simulink model "Simulation"  (R2022b)
settings: Solver=FixedStepAuto  StartTime=0.0  StopTime=param.Tsim  FixedStep=param.tSample  RelTol=1e-3
StopFcn:
  | run animation
  | run plotSol
undefined symbols (not defined in the file or in its folder): f, filterFr, filterFw, filterMr, FR_neg, FR_pos, g1, g2, g3, kFr, ki, kiSeil, kMr, kp, kpSeil, kVSl, kVSx, MR, MRP, param, xi_0
libraries: simulink x10, spsFirstOrderFilterLib x2
(part 2 of 3)

== system Simulation/Flatness-based control1/dynamic tracking control/Computation of the flat output ==
  Control input : Inport
  States : Inport  Port=2
  Demux : Demux  Outputs=8
  Demux1 : Demux  Outputs=2
  Derivative : Derivative
  Derivative1 : Derivative
  MATLAB Function : MATLAB Function  TreatAsAtomicUnit=on
  MATLAB Function1 : MATLAB Function  TreatAsAtomicUnit=on
  MATLAB Function2 : MATLAB Function  TreatAsAtomicUnit=on
  Mux : Mux
  Mux1 : Mux
  z1_xLoad : Outport
  z2_yLoad : Outport  Port=2
  wires:
  MATLAB Function/2(z2) -> Mux1/1
  Derivative/1 -> Mux/4
  MATLAB Function2/1(ddz1) -> Mux/3, Derivative/1
  MATLAB Function/1(z1) -> Mux/1
  Demux/2 -> MATLAB Function1/1(x2)
  Demux/6 -> MATLAB Function2/3(x6), MATLAB Function1/5(x6)
  MATLAB Function2/2(ddz2) -> Mux1/3, Derivative1/1
  Control input/1 -> Demux1/1
  MATLAB Function1/2(dz2) -> Mux1/2
  Demux/5 -> MATLAB Function/3(x5), MATLAB Function2/2(x5), MATLAB Function1/4(x5)
  Demux/1 -> MATLAB Function/1(x1)
  States/1 -> Demux/1
  Demux/3 -> MATLAB Function2/1(x3), MATLAB Function1/2(x3), MATLAB Function/2(x3)
  Demux/4 -> MATLAB Function1/3(x4)
  MATLAB Function1/1(dz1) -> Mux/2
  Derivative1/1 -> Mux1/4
  Mux/1 -> z1_xLoad/1
  Mux1/1 -> z2_yLoad/1
  Demux1/1 -> MATLAB Function2/4(u1)
  Demux1/2 -> MATLAB Function2/5(u2)

== system Simulation/Flatness-based control1/dynamic tracking control/System extension ==
  u_extended : Inport
  x_real : Inport  Port=2
  Demux : Demux  Outputs=6
  Demux1 : Demux  Outputs=2
  Integrator : Integrator
  Integrator1 : Integrator
  MATLAB Function3 : MATLAB Function  TreatAsAtomicUnit=on
  Mux : Mux  Inputs=8
  u2_real : Outport
  x_extended : Outport  Port=2
  wires:
  u_extended/1 -> Demux1/1
  x_real/1 -> Demux/1
  Mux/1 -> x_extended/1
  Demux/1 -> Mux/1
  Demux1/1 -> MATLAB Function3/5(u1_ext), Mux/2
  Demux/3 -> Mux/3, MATLAB Function3/2(x3)
  MATLAB Function3/1(u2_real) -> Mux/4, u2_real/1
  Demux/5 -> MATLAB Function3/3(x5), Mux/5
  Demux/6 -> Mux/6, MATLAB Function3/4(x6)
  Demux1/2 -> Integrator/1
  Integrator/1 -> Mux/8, Integrator1/1  "x2_ext"
  Integrator1/1 -> Mux/7, MATLAB Function3/1(x1_ext)  "x1_ext"

== system Simulation/Flatness-based control1/dynamic tracking control/Tracking controller ==
  z1_xLoad : Inport
  z2_yLoad : Inport  Port=2
  z1_d_xLoad : Inport  Port=3
  z2_d_yLoad : Inport  Port=4
  Constant : Constant  Value=[param.pX01 param.pX02 param.pX03 param.pX04]
  Constant1 : Constant  Value=[param.pY01_DYN param.pY02_DYN param.pY03_DYN param.pY04_DYN]
  Demux : Demux
  Demux1 : Demux
  MATLAB Function : MATLAB Function  TreatAsAtomicUnit=on
  Tracking controller v1 for xLoad : Subsystem
  Tracking controller v2 for yLoad : Subsystem
  u1_aCart : Outport
  u2_aRope : Outport  Port=2
  wires:
  Constant1/1 -> Tracking controller v2 for yLoad/3(Koeffizienten2)
  Constant/1 -> Tracking controller v1 for xLoad/3(Koeffizienten1)
  z2_d_yLoad/1 -> Tracking controller v2 for yLoad/1(z2_soll)
  z1_d_xLoad/1 -> Tracking controller v1 for xLoad/1(z1_soll)
  z1_xLoad/1 -> Demux/1, Tracking controller v1 for xLoad/2(z1_ist)
  MATLAB Function/2(u2) -> u2_aRope/1
  Demux1/1 -> MATLAB Function/4(z2)
  Demux/4 -> MATLAB Function/2(dddz1)
  z2_yLoad/1 -> Demux1/1, Tracking controller v2 for yLoad/2(z2_ist)
  Demux1/2 -> MATLAB Function/5(dz2)
  Tracking controller v1 for xLoad/1(v1) -> MATLAB Function/3(v1)
  MATLAB Function/1(u1) -> u1_aCart/1
  Demux/3 -> MATLAB Function/1(ddz1)
  Tracking controller v2 for yLoad/1(v2) -> MATLAB Function/8(v2)
  Demux1/3 -> MATLAB Function/6(ddz2)
  Demux1/4 -> MATLAB Function/7(dddz2)

== system Simulation/Flatness-based control1/quasistatic tracking control/Computation of the flat output ==
  Control input : Inport
  States : Inport  Port=2
  Demux : Demux  Outputs=6
  Demux1 : Demux  Outputs=2
  Derivative : Derivative
  Derivative1 : Derivative
  MATLAB Function : MATLAB Function  TreatAsAtomicUnit=on
  MATLAB Function1 : MATLAB Function  TreatAsAtomicUnit=on
  MATLAB Function2 : MATLAB Function  TreatAsAtomicUnit=on
  Mux : Mux
  Mux1 : Mux
  z1_xLoad : Outport
  z2_yLoad : Outport  Port=2
  wires:
  States/1 -> Demux/1
  Demux/1 -> MATLAB Function/1(x1)
  Demux/3 -> MATLAB Function2/1(x3), MATLAB Function1/2(x3), MATLAB Function/2(x3)
  Demux/5 -> MATLAB Function/3(x5), MATLAB Function2/2(x5), MATLAB Function1/4(x5)
  Control input/1 -> Demux1/1
  Mux1/1 -> z2_yLoad/1
  Mux/1 -> z1_xLoad/1
  Demux/2 -> MATLAB Function1/1(x2)
  Demux/4 -> MATLAB Function1/3(x4)
  Demux/6 -> MATLAB Function2/3(x6), MATLAB Function1/5(x6)
  Demux1/1 -> MATLAB Function2/4(u1)
  Demux1/2 -> MATLAB Function2/5(u2)
  MATLAB Function2/1(ddz1) -> Mux/3, Derivative/1
  MATLAB Function2/2(ddz2) -> Mux1/3, Derivative1/1
  Derivative/1 -> Mux/4
  Derivative1/1 -> Mux1/4
  MATLAB Function1/2(dz2) -> Mux1/2
  MATLAB Function/2(z2) -> Mux1/1
  MATLAB Function/1(z1) -> Mux/1
  MATLAB Function1/1(dz1) -> Mux/2

== system Simulation/Flatness-based control1/quasistatic tracking control/Tracking controller ==
  z1_xLoad : Inport
  z2_yLoad : Inport  Port=2
  z1_d_xLoad : Inport  Port=3
  z2_d_yLoad : Inport  Port=4
  Constant : Constant  Value=[param.pX01 param.pX02 param.pX03 param.pX04]
  Constant1 : Constant  Value=[param.pY01_QS param.pY02_QS]
  Demux : Demux
  Demux1 : Demux
  MATLAB Function : MATLAB Function  TreatAsAtomicUnit=on
  Tracking controller v1 for xLoad : Subsystem
  Tracking controller v2 for yLoad : Subsystem
  u1_aCart : Outport
  u2_aRope : Outport  Port=2
  wires:
  Constant1/1 -> Tracking controller v2 for yLoad/3(Koeffizienten2)
  Constant/1 -> Tracking controller v1 for xLoad/3(Koeffizienten1)
  z2_yLoad/1 -> Demux1/1, Tracking controller v2 for yLoad/2(z2_ist)
  z2_d_yLoad/1 -> Tracking controller v2 for yLoad/1(z2_soll)
  z1_xLoad/1 -> Demux/1, Tracking controller v1 for xLoad/2(z1_ist)
  z1_d_xLoad/1 -> Tracking controller v1 for xLoad/1(z1_soll)
  MATLAB Function/1(u1) -> u1_aCart/1
  MATLAB Function/2(u2) -> u2_aRope/1
  Tracking controller v2 for yLoad/3(ddv2) -> MATLAB Function/8(ddv2)
  Tracking controller v2 for yLoad/2(dv2) -> MATLAB Function/7(dv2)
  Tracking controller v2 for yLoad/1(v2) -> MATLAB Function/6(v2)
  Tracking controller v1 for xLoad/1(v1) -> MATLAB Function/3(v1)
  Demux/4 -> MATLAB Function/2(dddz1)
  Demux/3 -> MATLAB Function/1(ddz1)
  Demux1/1 -> MATLAB Function/4(z2)
  Demux1/2 -> MATLAB Function/5(dz2)

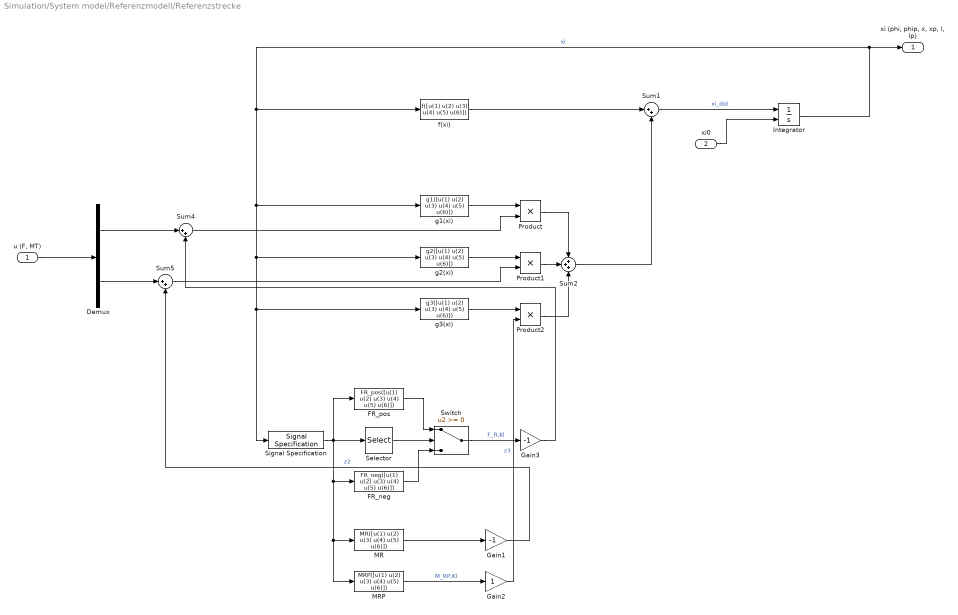
== system Simulation/System model/Referenzmodell/Referenzstrecke ==
  "u (F, MT)" : Inport
  xi0 : Inport  Port=2
  Demux : Demux  Outputs=2
  FR_neg : MATLABFcn  MATLABFcn=FR_neg([u(1) u(2) u(3) u(4) u(5) u(6)])
  FR_pos : MATLABFcn  MATLABFcn=FR_pos([u(1) u(2) u(3) u(4) u(5) u(6)])
  Gain1 : Gain  Gain=-1
  Gain2 : Gain
  Gain3 : Gain  Gain=-1
  Integrator : Integrator  InitialConditionSource=external  InitialCondition=xi_0
  MR : MATLABFcn  MATLABFcn=MR([u(1) u(2) u(3) u(4) u(5) u(6)])
  MRP : MATLABFcn  MATLABFcn=MRP([u(1) u(2) u(3) u(4) u(5) u(6)])
  Product : Product  RndMeth=Zero
  Product1 : Product  RndMeth=Zero
  Product2 : Product  RndMeth=Zero
  Selector : Selector  InputPortWidth=6  IndexOptions=Index vector (dialog)  Indices=4  OutputSizes=1
  Signal Specification : SignalSpecification  Dimensions=6
  Sum1 : Sum  Inputs=|++
  Sum2 : Sum  Inputs=+++
  Sum4 : Sum  Inputs=|++
  Sum5 : Sum  Inputs=|++
  Switch : Switch  ZeroCross=off  SaturateOnIntegerOverflow=off  InputSameDT=off
  f(xi) : MATLABFcn  MATLABFcn=f([u(1) u(2) u(3) u(4) u(5) u(6)])
  g1(xi) : MATLABFcn  MATLABFcn=g1([u(1) u(2) u(3) u(4) u(5) u(6)])
  g2(xi) : MATLABFcn  MATLABFcn=g2([u(1) u(2) u(3) u(4) u(5) u(6)])
  g3(xi) : MATLABFcn  MATLABFcn=g3([u(1) u(2) u(3) u(4) u(5) u(6)])
  "xi (phi, phip, x, xp, l, lp)" : Outport  VectorParamsAs1DForOutWhenUnconnected=off
  wires:
  Sum1/1 -> Integrator/1  "xi_dot"
  f(xi)/1 -> Sum1/1
  Product/1 -> Sum2/1
  Product1/1 -> Sum2/2
  Product2/1 -> Sum2/3
  Sum2/1 -> Sum1/2
  "u (F, MT)"/1 -> Demux/1
  Integrator/1 -> Signal Specification/1, g3(xi)/1, g2(xi)/1, g1(xi)/1, f(xi)/1, "xi (phi, phip, x, xp, l, lp)"/1  "xi"
  FR_pos/1 -> Switch/1
  Selector/1 -> Switch/2
  FR_neg/1 -> Switch/3
  MRP/1 -> Gain2/1  "M_RP,Kl"
  Switch/1 -> Gain3/1  "F_R,Kl"
  Gain1/1 -> Sum5/2  "z2"
  Gain2/1 -> Product2/2  "z3"
  Demux/1 -> Sum4/1
  Sum4/1 -> Product/2
  Demux/2 -> Sum5/1
  Sum5/1 -> Product1/2
  xi0/1 -> Integrator/2
  g1(xi)/1 -> Product/1
  g2(xi)/1 -> Product1/1
  g3(xi)/1 -> Product2/1
  MR/1 -> Gain1/1
  Gain3/1 -> Sum4/2
  Signal Specification/1 -> FR_neg/1, MR/1, MRP/1, FR_pos/1, Selector/1

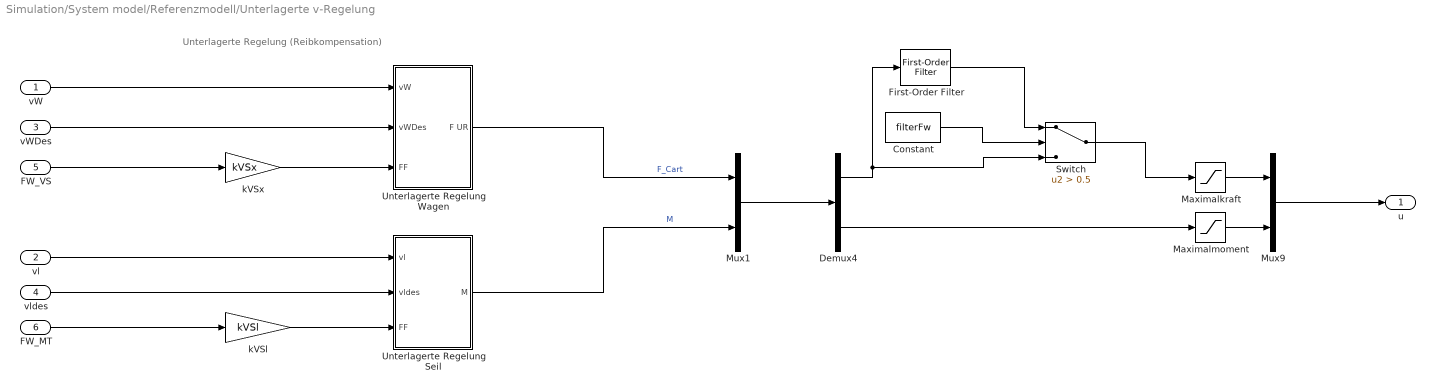
== system Simulation/System model/Referenzmodell/Unterlagerte v-Regelung ==
  note: Unterlagerte Regelung (Reibkompensation)
  vW : Inport
  vl : Inport  Port=2
  vWDes : Inport  Port=3
  vldes : Inport  Port=4
  FW_VS : Inport  Port=5
  FW_MT : Inport  Port=6
  Constant : Constant  Value=filterFw
  Demux4 : Demux  Outputs=2
  First-Order Filter : spsFirstOrderFilterLib/First-Order Filter  FilterType=Lowpass  Tc=filterFwT  Ts=param.tSample  Initialize=on  Vac_Init=[0, 0, 60]  Vdc_Init=0  PlotResponse=off  FreqRange="[0,  200,  1]"
  Maximalkraft : Saturate  UpperLimit=param.ScaleFmax*param.Fmax  LowerLimit=-param.ScaleFmax*param.Fmax
  Maximalmoment : Saturate  UpperLimit=param.M_Tmax  LowerLimit=-param.M_Tmax
  Mux1 : Mux  Inputs=2
  Mux9 : Mux  Inputs=2
  Switch : Switch  Criteria=u2 > Threshold  Threshold=0.5  SaturateOnIntegerOverflow=off  InputSameDT=off
  Unterlagerte Regelung Seil : Subsystem
  Unterlagerte Regelung Wagen : Subsystem
  kVSl : Gain  Gain=kVSl
  kVSx : Gain  Gain=kVSx
  u : Outport  PortDimensions=2  VectorParamsAs1DForOutWhenUnconnected=off
  wires:
  Demux4/2 -> Maximalmoment/1
  Mux1/1 -> Demux4/1
  Maximalmoment/1 -> Mux9/2
  kVSl/1 -> Unterlagerte Regelung Seil/3(FF)
  kVSx/1 -> Unterlagerte Regelung Wagen/3(FF)
  Demux4/1 -> First-Order Filter/1, Switch/3
  Mux9/1 -> u/1
  Unterlagerte Regelung Wagen/1(F UR) -> Mux1/1  "F_Cart"
  Unterlagerte Regelung Seil/1(M) -> Mux1/2  "M"
  Maximalkraft/1 -> Mux9/1
  vW/1 -> Unterlagerte Regelung Wagen/1(vW)
  FW_VS/1 -> kVSx/1
  vl/1 -> Unterlagerte Regelung Seil/1(vl)
  vldes/1 -> Unterlagerte Regelung Seil/2(vldes)
  FW_MT/1 -> kVSl/1
  vWDes/1 -> Unterlagerte Regelung Wagen/2(vWDes)
  Constant/1 -> Switch/2
  First-Order Filter/1 -> Switch/1
  Switch/1 -> Maximalkraft/1

== system Simulation/System model/Referenzmodell/Vorsteuerung Trommel ==
  aS : Inport
  Constant3 : Constant  Value=-param.J
  Constant5 : Constant  Value=(1/param.rho)
  Product1 : Product
  Product2 : Product
  FF MT : Outport  VectorParamsAs1DForOutWhenUnconnected=off
  wires:
  Constant3/1 -> Product1/1
  Product2/1 -> Product1/2
  Constant5/1 -> Product2/1
  aS/1 -> Product2/2
  Product1/1 -> FF MT/1

== system Simulation/System model/Referenzmodell/Vorsteuerung Wagen ==
  aW : Inport
  Constant2 : Constant  Value=param.m1
  Product : Product
  FF FW : Outport  VectorParamsAs1DForOutWhenUnconnected=off
  wires:
  Product/1 -> FF FW/1
  Constant2/1 -> Product/1
  aW/1 -> Product/2

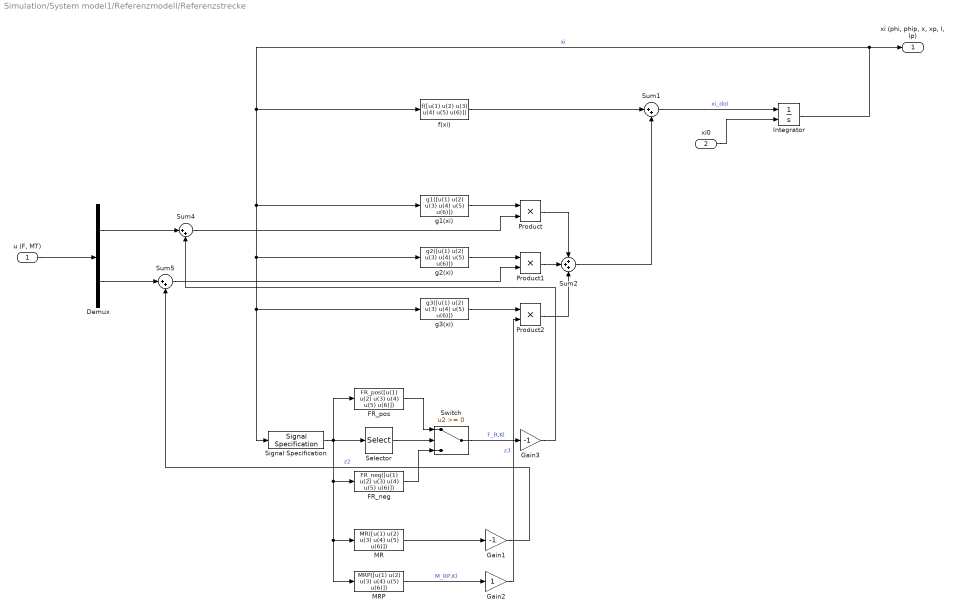
== system Simulation/System model1/Referenzmodell/Referenzstrecke ==
  "u (F, MT)" : Inport
  xi0 : Inport  Port=2
  Demux : Demux  Outputs=2
  FR_neg : MATLABFcn  MATLABFcn=FR_neg([u(1) u(2) u(3) u(4) u(5) u(6)])
  FR_pos : MATLABFcn  MATLABFcn=FR_pos([u(1) u(2) u(3) u(4) u(5) u(6)])
  Gain1 : Gain  Gain=-1
  Gain2 : Gain
  Gain3 : Gain  Gain=-1
  Integrator : Integrator  InitialConditionSource=external  InitialCondition=xi_0
  MR : MATLABFcn  MATLABFcn=MR([u(1) u(2) u(3) u(4) u(5) u(6)])
  MRP : MATLABFcn  MATLABFcn=MRP([u(1) u(2) u(3) u(4) u(5) u(6)])
  Product : Product  RndMeth=Zero
  Product1 : Product  RndMeth=Zero
  Product2 : Product  RndMeth=Zero
  Selector : Selector  InputPortWidth=6  IndexOptions=Index vector (dialog)  Indices=4  OutputSizes=1
  Signal Specification : SignalSpecification  Dimensions=6
  Sum1 : Sum  Inputs=|++
  Sum2 : Sum  Inputs=+++
  Sum4 : Sum  Inputs=|++
  Sum5 : Sum  Inputs=|++
  Switch : Switch  ZeroCross=off  SaturateOnIntegerOverflow=off  InputSameDT=off
  f(xi) : MATLABFcn  MATLABFcn=f([u(1) u(2) u(3) u(4) u(5) u(6)])
  g1(xi) : MATLABFcn  MATLABFcn=g1([u(1) u(2) u(3) u(4) u(5) u(6)])
  g2(xi) : MATLABFcn  MATLABFcn=g2([u(1) u(2) u(3) u(4) u(5) u(6)])
  g3(xi) : MATLABFcn  MATLABFcn=g3([u(1) u(2) u(3) u(4) u(5) u(6)])
  "xi (phi, phip, x, xp, l, lp)" : Outport  VectorParamsAs1DForOutWhenUnconnected=off
  wires:
  Sum1/1 -> Integrator/1  "xi_dot"
  f(xi)/1 -> Sum1/1
  Product/1 -> Sum2/1
  Product1/1 -> Sum2/2
  Product2/1 -> Sum2/3
  Sum2/1 -> Sum1/2
  "u (F, MT)"/1 -> Demux/1
  Integrator/1 -> Signal Specification/1, g3(xi)/1, g2(xi)/1, g1(xi)/1, f(xi)/1, "xi (phi, phip, x, xp, l, lp)"/1  "xi"
  FR_pos/1 -> Switch/1
  Selector/1 -> Switch/2
  FR_neg/1 -> Switch/3
  MRP/1 -> Gain2/1  "M_RP,Kl"
  Switch/1 -> Gain3/1  "F_R,Kl"
  Gain1/1 -> Sum5/2  "z2"
  Gain2/1 -> Product2/2  "z3"
  Demux/1 -> Sum4/1
  Sum4/1 -> Product/2
  Demux/2 -> Sum5/1
  Sum5/1 -> Product1/2
  xi0/1 -> Integrator/2
  g1(xi)/1 -> Product/1
  g2(xi)/1 -> Product1/1
  g3(xi)/1 -> Product2/1
  MR/1 -> Gain1/1
  Gain3/1 -> Sum4/2
  Signal Specification/1 -> FR_neg/1, MR/1, MRP/1, FR_pos/1, Selector/1

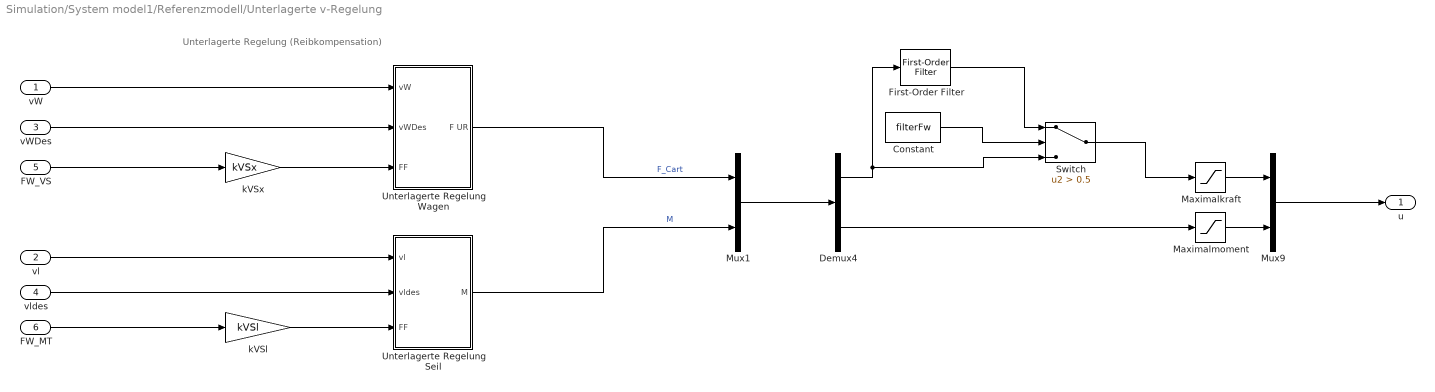
== system Simulation/System model1/Referenzmodell/Unterlagerte v-Regelung ==
  note: Unterlagerte Regelung (Reibkompensation)
  vW : Inport
  vl : Inport  Port=2
  vWDes : Inport  Port=3
  vldes : Inport  Port=4
  FW_VS : Inport  Port=5
  FW_MT : Inport  Port=6
  Constant : Constant  Value=filterFw
  Demux4 : Demux  Outputs=2
  First-Order Filter : spsFirstOrderFilterLib/First-Order Filter  FilterType=Lowpass  Tc=filterFwT  Ts=param.tSample  Initialize=on  Vac_Init=[0, 0, 60]  Vdc_Init=0  PlotResponse=off  FreqRange="[0,  200,  1]"
  Maximalkraft : Saturate  UpperLimit=param.ScaleFmax*param.Fmax  LowerLimit=-param.ScaleFmax*param.Fmax
  Maximalmoment : Saturate  UpperLimit=param.M_Tmax  LowerLimit=-param.M_Tmax
  Mux1 : Mux  Inputs=2
  Mux9 : Mux  Inputs=2
  Switch : Switch  Criteria=u2 > Threshold  Threshold=0.5  SaturateOnIntegerOverflow=off  InputSameDT=off
  Unterlagerte Regelung Seil : Subsystem
  Unterlagerte Regelung Wagen : Subsystem
  kVSl : Gain  Gain=kVSl
  kVSx : Gain  Gain=kVSx
  u : Outport  PortDimensions=2  VectorParamsAs1DForOutWhenUnconnected=off
  wires:
  Demux4/2 -> Maximalmoment/1
  Mux1/1 -> Demux4/1
  Maximalmoment/1 -> Mux9/2
  kVSl/1 -> Unterlagerte Regelung Seil/3(FF)
  kVSx/1 -> Unterlagerte Regelung Wagen/3(FF)
  Demux4/1 -> First-Order Filter/1, Switch/3
  Mux9/1 -> u/1
  Unterlagerte Regelung Wagen/1(F UR) -> Mux1/1  "F_Cart"
  Unterlagerte Regelung Seil/1(M) -> Mux1/2  "M"
  Maximalkraft/1 -> Mux9/1
  vW/1 -> Unterlagerte Regelung Wagen/1(vW)
  FW_VS/1 -> kVSx/1
  vl/1 -> Unterlagerte Regelung Seil/1(vl)
  vldes/1 -> Unterlagerte Regelung Seil/2(vldes)
  FW_MT/1 -> kVSl/1
  vWDes/1 -> Unterlagerte Regelung Wagen/2(vWDes)
  Constant/1 -> Switch/2
  First-Order Filter/1 -> Switch/1
  Switch/1 -> Maximalkraft/1

== system Simulation/System model1/Referenzmodell/Vorsteuerung Trommel ==
  aS : Inport
  Constant3 : Constant  Value=-param.J
  Constant5 : Constant  Value=(1/param.rho)
  Product1 : Product
  Product2 : Product
  FF MT : Outport  VectorParamsAs1DForOutWhenUnconnected=off
  wires:
  Constant3/1 -> Product1/1
  Product2/1 -> Product1/2
  Constant5/1 -> Product2/1
  aS/1 -> Product2/2
  Product1/1 -> FF MT/1

== system Simulation/System model1/Referenzmodell/Vorsteuerung Wagen ==
  aW : Inport
  Constant2 : Constant  Value=param.m1
  Product : Product
  FF FW : Outport  VectorParamsAs1DForOutWhenUnconnected=off
  wires:
  Product/1 -> FF FW/1
  Constant2/1 -> Product/1
  aW/1 -> Product/2

== system Simulation/Flatness-based control/dynamic tracking control/Tracking controller/Tracking controller v1 for xLoad ==
  z1_soll : Inport
  z1_ist : Inport  Port=2
  Koeffizienten1 : Inport  Port=3
  Demux : Demux
  Demux1 : Demux
  Demux2 : Demux
  Derivative : Derivative
  MATLAB Function : MATLAB Function  TreatAsAtomicUnit=on
  v1 : Outport
  wires:
  MATLAB Function/1(v1) -> v1/1
  Demux1/2 -> MATLAB Function/7(dz1)
  Demux/4 -> Derivative/1, MATLAB Function/4(dddz1_star)
  Demux/3 -> MATLAB Function/3(ddz1_star)
  Demux1/4 -> MATLAB Function/9(dddz1)
  Demux2/3 -> MATLAB Function/12(pX03)
  Demux2/4 -> MATLAB Function/13(pX04)
  z1_soll/1 -> Demux/1
  Derivative/1 -> MATLAB Function/5(d4z1_star)
  Demux2/2 -> MATLAB Function/11(pX02)
  Demux2/1 -> MATLAB Function/10(pX01)
  Demux1/3 -> MATLAB Function/8(ddz1)
  Koeffizienten1/1 -> Demux2/1
  Demux/1 -> MATLAB Function/1(z1_star)
  Demux/2 -> MATLAB Function/2(dz1_star)
  z1_ist/1 -> Demux1/1
  Demux1/1 -> MATLAB Function/6(z1)

== system Simulation/Flatness-based control/dynamic tracking control/Tracking controller/Tracking controller v2 for yLoad ==
  z2_soll : Inport
  z2_ist : Inport  Port=2
  Koeffizienten2 : Inport  Port=3
  Demux : Demux
  Demux1 : Demux
  Demux2 : Demux
  Derivative : Derivative
  MATLAB Function : MATLAB Function  TreatAsAtomicUnit=on
  v2 : Outport
  wires:
  MATLAB Function/1(v1) -> v2/1
  Demux1/2 -> MATLAB Function/7(dz1)
  Demux/4 -> Derivative/1, MATLAB Function/4(dddz1_star)
  Demux/3 -> MATLAB Function/3(ddz1_star)
  Demux1/4 -> MATLAB Function/9(dddz1)
  Demux2/3 -> MATLAB Function/12(pY03_DYN)
  Demux2/4 -> MATLAB Function/13(pY04_DYN)
  z2_soll/1 -> Demux/1
  Derivative/1 -> MATLAB Function/5(d4z1_star)
  Demux2/2 -> MATLAB Function/11(pY02_DYN)
  Demux2/1 -> MATLAB Function/10(pY01_DYN)
  Demux1/3 -> MATLAB Function/8(ddz1)
  Koeffizienten2/1 -> Demux2/1
  Demux/1 -> MATLAB Function/1(z1_star)
  Demux/2 -> MATLAB Function/2(dz1_star)
  z2_ist/1 -> Demux1/1
  Demux1/1 -> MATLAB Function/6(z1)

== system Simulation/Flatness-based control/quasistatic tracking control/Tracking controller/Tracking controller v1 for xLoad ==
  z1_soll : Inport
  z1_ist : Inport  Port=2
  Koeffizienten1 : Inport  Port=3
  Demux : Demux
  Demux1 : Demux
  Demux2 : Demux
  Derivative : Derivative
  MATLAB Function : MATLAB Function  TreatAsAtomicUnit=on
  v1 : Outport
  wires:
  z1_soll/1 -> Demux/1
  z1_ist/1 -> Demux1/1
  Koeffizienten1/1 -> Demux2/1
  Demux2/1 -> MATLAB Function/10(pX01)
  Demux2/2 -> MATLAB Function/11(pX02)
  Demux2/3 -> MATLAB Function/12(pX03)
  Demux2/4 -> MATLAB Function/13(pX04)
  Demux/1 -> MATLAB Function/1(z1_star)
  Demux/2 -> MATLAB Function/2(dz1_star)
  Demux/3 -> MATLAB Function/3(ddz1_star)
  Demux/4 -> Derivative/1, MATLAB Function/4(dddz1_star)
  Demux1/1 -> MATLAB Function/6(z1)
  Demux1/2 -> MATLAB Function/7(dz1)
  Demux1/3 -> MATLAB Function/8(ddz1)
  Demux1/4 -> MATLAB Function/9(dddz1)
  Derivative/1 -> MATLAB Function/5(d4z1_star)
  MATLAB Function/1(v1) -> v1/1

== system Simulation/Flatness-based control/quasistatic tracking control/Tracking controller/Tracking controller v2 for yLoad ==
  z2_soll : Inport
  z2_ist : Inport  Port=2
  Koeffizienten2 : Inport  Port=3
  Demux : Demux
  Demux1 : Demux
  Demux2 : Demux  Outputs=2
  Derivative : Derivative
  MATLAB Function : MATLAB Function  TreatAsAtomicUnit=on
  v2 : Outport
  dv2 : Outport  Port=2
  ddv2 : Outport  Port=3
  wires:
  MATLAB Function/1(v2) -> v2/1
  Demux1/2 -> MATLAB Function/7(dz2)
  Demux/4 -> Derivative/1, MATLAB Function/4(dddz2_star)
  Demux/3 -> MATLAB Function/3(ddz2_star)
  z2_soll/1 -> Demux/1
  Derivative/1 -> MATLAB Function/5(d4z2_star)
  Demux2/2 -> MATLAB Function/9(pY02_QS)
  Demux2/1 -> MATLAB Function/8(pY01_QS)
  Koeffizienten2/1 -> Demux2/1
  Demux/1 -> MATLAB Function/1(z2_star)
  Demux/2 -> MATLAB Function/2(dz2_star)
  z2_ist/1 -> Demux1/1
  Demux1/1 -> MATLAB Function/6(z2)
  MATLAB Function/2(dv2) -> dv2/1
  MATLAB Function/3(ddv2) -> ddv2/1

== system Simulation/Flatness-based control1/dynamic tracking control/Tracking controller/Tracking controller v1 for xLoad ==
  z1_soll : Inport
  z1_ist : Inport  Port=2
  Koeffizienten1 : Inport  Port=3
  Demux : Demux
  Demux1 : Demux
  Demux2 : Demux
  Derivative : Derivative
  MATLAB Function : MATLAB Function  TreatAsAtomicUnit=on
  v1 : Outport
  wires:
  MATLAB Function/1(v1) -> v1/1
  Demux1/2 -> MATLAB Function/7(dz1)
  Demux/4 -> Derivative/1, MATLAB Function/4(dddz1_star)
  Demux/3 -> MATLAB Function/3(ddz1_star)
  Demux1/4 -> MATLAB Function/9(dddz1)
  Demux2/3 -> MATLAB Function/12(pX03)
  Demux2/4 -> MATLAB Function/13(pX04)
  z1_soll/1 -> Demux/1
  Derivative/1 -> MATLAB Function/5(d4z1_star)
  Demux2/2 -> MATLAB Function/11(pX02)
  Demux2/1 -> MATLAB Function/10(pX01)
  Demux1/3 -> MATLAB Function/8(ddz1)
  Koeffizienten1/1 -> Demux2/1
  Demux/1 -> MATLAB Function/1(z1_star)
  Demux/2 -> MATLAB Function/2(dz1_star)
  z1_ist/1 -> Demux1/1
  Demux1/1 -> MATLAB Function/6(z1)

== system Simulation/Flatness-based control1/dynamic tracking control/Tracking controller/Tracking controller v2 for yLoad ==
  z2_soll : Inport
  z2_ist : Inport  Port=2
  Koeffizienten2 : Inport  Port=3
  Demux : Demux
  Demux1 : Demux
  Demux2 : Demux
  Derivative : Derivative
  MATLAB Function : MATLAB Function  TreatAsAtomicUnit=on
  v2 : Outport
  wires:
  MATLAB Function/1(v1) -> v2/1
  Demux1/2 -> MATLAB Function/7(dz1)
  Demux/4 -> Derivative/1, MATLAB Function/4(dddz1_star)
  Demux/3 -> MATLAB Function/3(ddz1_star)
  Demux1/4 -> MATLAB Function/9(dddz1)
  Demux2/3 -> MATLAB Function/12(pY03_DYN)
  Demux2/4 -> MATLAB Function/13(pY04_DYN)
  z2_soll/1 -> Demux/1
  Derivative/1 -> MATLAB Function/5(d4z1_star)
  Demux2/2 -> MATLAB Function/11(pY02_DYN)
  Demux2/1 -> MATLAB Function/10(pY01_DYN)
  Demux1/3 -> MATLAB Function/8(ddz1)
  Koeffizienten2/1 -> Demux2/1
  Demux/1 -> MATLAB Function/1(z1_star)
  Demux/2 -> MATLAB Function/2(dz1_star)
  z2_ist/1 -> Demux1/1
  Demux1/1 -> MATLAB Function/6(z1)

== system Simulation/Flatness-based control1/quasistatic tracking control/Tracking controller/Tracking controller v1 for xLoad ==
  z1_soll : Inport
  z1_ist : Inport  Port=2
  Koeffizienten1 : Inport  Port=3
  Demux : Demux
  Demux1 : Demux
  Demux2 : Demux
  Derivative : Derivative
  MATLAB Function : MATLAB Function  TreatAsAtomicUnit=on
  v1 : Outport
  wires:
  z1_soll/1 -> Demux/1
  z1_ist/1 -> Demux1/1
  Koeffizienten1/1 -> Demux2/1
  Demux2/1 -> MATLAB Function/10(pX01)
  Demux2/2 -> MATLAB Function/11(pX02)
  Demux2/3 -> MATLAB Function/12(pX03)
  Demux2/4 -> MATLAB Function/13(pX04)
  Demux/1 -> MATLAB Function/1(z1_star)
  Demux/2 -> MATLAB Function/2(dz1_star)
  Demux/3 -> MATLAB Function/3(ddz1_star)
  Demux/4 -> Derivative/1, MATLAB Function/4(dddz1_star)
  Demux1/1 -> MATLAB Function/6(z1)
  Demux1/2 -> MATLAB Function/7(dz1)
  Demux1/3 -> MATLAB Function/8(ddz1)
  Demux1/4 -> MATLAB Function/9(dddz1)
  Derivative/1 -> MATLAB Function/5(d4z1_star)
  MATLAB Function/1(v1) -> v1/1

== system Simulation/Flatness-based control1/quasistatic tracking control/Tracking controller/Tracking controller v2 for yLoad ==
  z2_soll : Inport
  z2_ist : Inport  Port=2
  Koeffizienten2 : Inport  Port=3
  Demux : Demux
  Demux1 : Demux
  Demux2 : Demux  Outputs=2
  Derivative : Derivative
  MATLAB Function : MATLAB Function  TreatAsAtomicUnit=on
  v2 : Outport
  dv2 : Outport  Port=2
  ddv2 : Outport  Port=3
  wires:
  MATLAB Function/1(v2) -> v2/1
  Demux1/2 -> MATLAB Function/7(dz2)
  Demux/4 -> Derivative/1, MATLAB Function/4(dddz2_star)
  Demux/3 -> MATLAB Function/3(ddz2_star)
  z2_soll/1 -> Demux/1
  Derivative/1 -> MATLAB Function/5(d4z2_star)
  Demux2/2 -> MATLAB Function/9(pY02_QS)
  Demux2/1 -> MATLAB Function/8(pY01_QS)
  Koeffizienten2/1 -> Demux2/1
  Demux/1 -> MATLAB Function/1(z2_star)
  Demux/2 -> MATLAB Function/2(dz2_star)
  z2_ist/1 -> Demux1/1
  Demux1/1 -> MATLAB Function/6(z2)
  MATLAB Function/2(dv2) -> dv2/1
  MATLAB Function/3(ddv2) -> ddv2/1

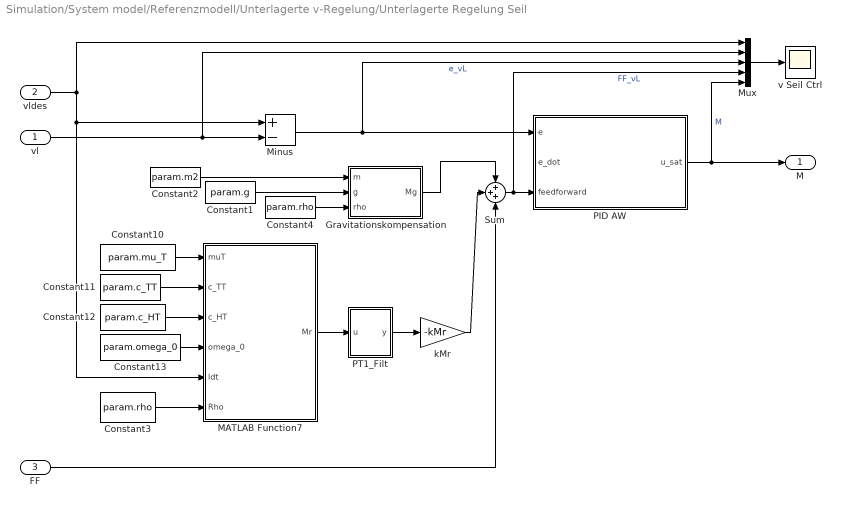
== system Simulation/System model/Referenzmodell/Unterlagerte v-Regelung/Unterlagerte Regelung Seil ==
  vl : Inport
  vldes : Inport  Port=2
  FF : Inport  Port=3
  Constant1 : Constant  Value=param.g
  Constant10 : Constant  Value=param.mu_T
  Constant11 : Constant  Value=param.c_TT
  Constant12 : Constant  Value=param.c_HT
  Constant13 : Constant  Value=param.omega_0
  Constant2 : Constant  Value=param.m2
  Constant3 : Constant  Value=param.rho
  Constant4 : Constant  Value=param.rho
  Gravitationskompensation : MATLAB Function  TreatAsAtomicUnit=on
  MATLAB Function7 : MATLAB Function  TreatAsAtomicUnit=on
  Minus : Sum  Inputs=+-
  Mux : Mux  Inputs=5
  PID AW : Subsystem  mask{K_P=kpSeil, K_I=kiSeil, K_D=0, u_max=param.M_Tmax, u_min=-param.M_Tmax}
      mask prompts: K_P "Proportional Gain"; K_I "Integrator Gain"; K_D "Derivative Gain"; u_max "Maximal Output"; u_min "Minimal Output"
      mask Display: disp('PID with Anti-Windup\n and external FF /\n additional input\n(c) by M. Lukassek')
  PT1_Filt : Subsystem
  Sum : Sum  Inputs=+++
  kMr : Gain  Gain=-kMr
  v Seil Ctrl : Scope
  M : Outport  PortDimensions=1  VectorParamsAs1DForOutWhenUnconnected=off
  wires:
  Minus/1 -> Mux/3, PID AW/1(e)  "e_vL"
  Constant10/1 -> MATLAB Function7/1(muT)
  Constant12/1 -> MATLAB Function7/3(c_HT)
  Constant11/1 -> MATLAB Function7/2(c_TT)
  Constant13/1 -> MATLAB Function7/4(omega_0)
  Constant3/1 -> MATLAB Function7/6(Rho)
  MATLAB Function7/1(Mr) -> PT1_Filt/1(u)
  Constant1/1 -> Gravitationskompensation/2(g)
  Constant4/1 -> Gravitationskompensation/3(rho)
  Constant2/1 -> Gravitationskompensation/1(m)
  Mux/1 -> v Seil Ctrl/1
  vl/1 -> Mux/2, Minus/2
  PID AW/1(u_sat) -> Mux/5, M/1  "M"
  Sum/1 -> PID AW/3(feedforward), Mux/4  "FF_vL"
  kMr/1 -> Sum/2
  FF/1 -> Sum/3
  Gravitationskompensation/1(Mg) -> Sum/1
  vldes/1 -> MATLAB Function7/5(ldt), Minus/1, Mux/1
  PT1_Filt/1(y) -> kMr/1

== system Simulation/System model/Referenzmodell/Unterlagerte v-Regelung/Unterlagerte Regelung Wagen ==
  vW : Inport
  vWDes : Inport  Port=2
  FF : Inport  Port=3
  Constant1 : Constant  Value=param.mu_W_pos
  Constant2 : Constant  Value=param.c_TW_pos
  Constant3 : Constant  Value=param.c_HW_pos
  Constant4 : Constant  Value=param.v_0_pos
  Dead Zone : DeadZone  LowerValue=-0.1  UpperValue=0.1
  MATLAB Function2 : MATLAB Function  TreatAsAtomicUnit=on
  Mux : Mux  Inputs=5
  PID AW : Subsystem  mask{K_P=kp, K_I=ki, K_D=0, u_max=param.ScaleFmax*param.Fmax, u_min=-param.ScaleFmax*param.Fmax}
      mask prompts: K_P "Proportional Gain"; K_I "Integrator Gain"; K_D "Derivative Gain"; u_max "Maximal Output"; u_min "Minimal Output"
      mask Display: disp('PID with Anti-Windup\n and external FF /\n additional input\n(c) by M. Lukassek')
  PT1_Filt : Subsystem
  Sum1 : Sum  Inputs=|+-  AccumDataTypeStr=double  OutDataTypeStr=double
  Sum2 : Sum  Inputs=|++  AccumDataTypeStr=double  OutDataTypeStr=double
  kFr : Gain  Gain=-kFr
  v Wagen Ctrl : Scope
  F UR : Outport  VectorParamsAs1DForOutWhenUnconnected=off
  wires:
  Sum1/1 -> Mux/3, PID AW/1(e)  "e_vW"
  PID AW/1(u_sat) -> Mux/4, F UR/1  "F"
  MATLAB Function2/1(Fr) -> PT1_Filt/1(u)
  Constant1/1 -> MATLAB Function2/1(mu_W_pos)
  Constant2/1 -> MATLAB Function2/2(c_TW_pos)
  Constant3/1 -> MATLAB Function2/3(c_HW_pos)
  Constant4/1 -> MATLAB Function2/4(v_0_pos)
  vW/1 -> Mux/2, Sum1/2
  Mux/1 -> v Wagen Ctrl/1
  Sum2/1 -> Mux/5, PID AW/3(feedforward)  "FF_vW"
  kFr/1 -> Sum2/1
  FF/1 -> Sum2/2
  vWDes/1 -> Mux/1, Sum1/1, Dead Zone/1
  Dead Zone/1 -> MATLAB Function2/5(xdt)
  PT1_Filt/1(y) -> kFr/1

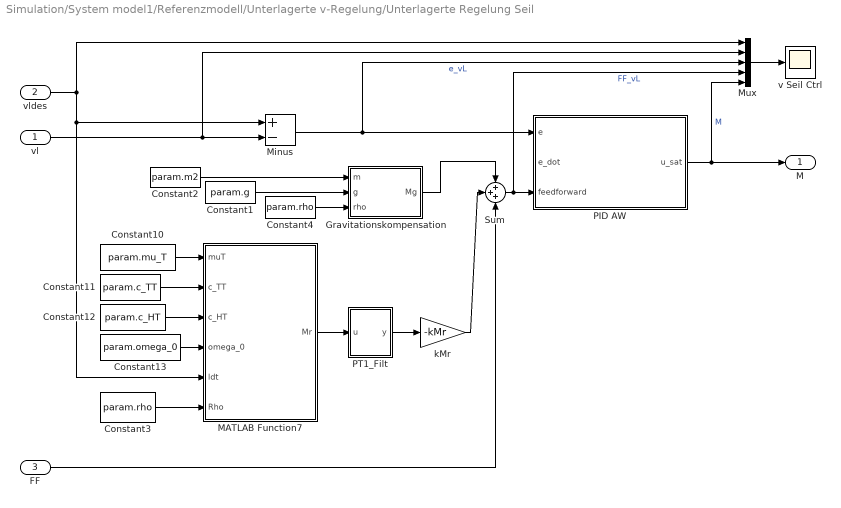
== system Simulation/System model1/Referenzmodell/Unterlagerte v-Regelung/Unterlagerte Regelung Seil ==
  vl : Inport
  vldes : Inport  Port=2
  FF : Inport  Port=3
  Constant1 : Constant  Value=param.g
  Constant10 : Constant  Value=param.mu_T
  Constant11 : Constant  Value=param.c_TT
  Constant12 : Constant  Value=param.c_HT
  Constant13 : Constant  Value=param.omega_0
  Constant2 : Constant  Value=param.m2
  Constant3 : Constant  Value=param.rho
  Constant4 : Constant  Value=param.rho
  Gravitationskompensation : MATLAB Function  TreatAsAtomicUnit=on
  MATLAB Function7 : MATLAB Function  TreatAsAtomicUnit=on
  Minus : Sum  Inputs=+-
  Mux : Mux  Inputs=5
  PID AW : Subsystem  mask{K_P=kpSeil, K_I=kiSeil, K_D=0, u_max=param.M_Tmax, u_min=-param.M_Tmax}
      mask prompts: K_P "Proportional Gain"; K_I "Integrator Gain"; K_D "Derivative Gain"; u_max "Maximal Output"; u_min "Minimal Output"
      mask Display: disp('PID with Anti-Windup\n and external FF /\n additional input\n(c) by M. Lukassek')
  PT1_Filt : Subsystem
  Sum : Sum  Inputs=+++
  kMr : Gain  Gain=-kMr
  v Seil Ctrl : Scope
  M : Outport  PortDimensions=1  VectorParamsAs1DForOutWhenUnconnected=off
  wires:
  Minus/1 -> Mux/3, PID AW/1(e)  "e_vL"
  Constant10/1 -> MATLAB Function7/1(muT)
  Constant12/1 -> MATLAB Function7/3(c_HT)
  Constant11/1 -> MATLAB Function7/2(c_TT)
  Constant13/1 -> MATLAB Function7/4(omega_0)
  Constant3/1 -> MATLAB Function7/6(Rho)
  MATLAB Function7/1(Mr) -> PT1_Filt/1(u)
  Constant1/1 -> Gravitationskompensation/2(g)
  Constant4/1 -> Gravitationskompensation/3(rho)
  Constant2/1 -> Gravitationskompensation/1(m)
  Mux/1 -> v Seil Ctrl/1
  vl/1 -> Mux/2, Minus/2
  PID AW/1(u_sat) -> Mux/5, M/1  "M"
  Sum/1 -> PID AW/3(feedforward), Mux/4  "FF_vL"
  kMr/1 -> Sum/2
  FF/1 -> Sum/3
  Gravitationskompensation/1(Mg) -> Sum/1
  vldes/1 -> MATLAB Function7/5(ldt), Minus/1, Mux/1
  PT1_Filt/1(y) -> kMr/1

== system Simulation/System model1/Referenzmodell/Unterlagerte v-Regelung/Unterlagerte Regelung Wagen ==
  vW : Inport
  vWDes : Inport  Port=2
  FF : Inport  Port=3
  Constant1 : Constant  Value=param.mu_W_pos
  Constant2 : Constant  Value=param.c_TW_pos
  Constant3 : Constant  Value=param.c_HW_pos
  Constant4 : Constant  Value=param.v_0_pos
  Dead Zone : DeadZone  LowerValue=-0.1  UpperValue=0.1
  MATLAB Function2 : MATLAB Function  TreatAsAtomicUnit=on
  Mux : Mux  Inputs=5
  PID AW : Subsystem  mask{K_P=kp, K_I=ki, K_D=0, u_max=param.ScaleFmax*param.Fmax, u_min=-param.ScaleFmax*param.Fmax}
      mask prompts: K_P "Proportional Gain"; K_I "Integrator Gain"; K_D "Derivative Gain"; u_max "Maximal Output"; u_min "Minimal Output"
      mask Display: disp('PID with Anti-Windup\n and external FF /\n additional input\n(c) by M. Lukassek')
  PT1_Filt : Subsystem
  Sum1 : Sum  Inputs=|+-  AccumDataTypeStr=double  OutDataTypeStr=double
  Sum2 : Sum  Inputs=|++  AccumDataTypeStr=double  OutDataTypeStr=double
  kFr : Gain  Gain=-kFr
  v Wagen Ctrl : Scope
  F UR : Outport  VectorParamsAs1DForOutWhenUnconnected=off
  wires:
  Sum1/1 -> Mux/3, PID AW/1(e)  "e_vW"
  PID AW/1(u_sat) -> Mux/4, F UR/1  "F"
  MATLAB Function2/1(Fr) -> PT1_Filt/1(u)
  Constant1/1 -> MATLAB Function2/1(mu_W_pos)
  Constant2/1 -> MATLAB Function2/2(c_TW_pos)
  Constant3/1 -> MATLAB Function2/3(c_HW_pos)
  Constant4/1 -> MATLAB Function2/4(v_0_pos)
  vW/1 -> Mux/2, Sum1/2
  Mux/1 -> v Wagen Ctrl/1
  Sum2/1 -> Mux/5, PID AW/3(feedforward)  "FF_vW"
  kFr/1 -> Sum2/1
  FF/1 -> Sum2/2
  vWDes/1 -> Mux/1, Sum1/1, Dead Zone/1
  Dead Zone/1 -> MATLAB Function2/5(xdt)
  PT1_Filt/1(y) -> kFr/1

== system Simulation/System model/Referenzmodell/Unterlagerte v-Regelung/Unterlagerte Regelung Seil/PID AW ==
  e : Inport
  e_dot : Inport  Port=2
  feedforward : Inport  Port=3
  Integrator : Integrator
  Kaw : Gain  Gain=sign(K_I)
  Kd : Gain  Gain=K_D
  Ki : Gain  Gain=K_I
  Kp : Gain  Gain=K_P
  Saturation : Saturate  UpperLimit=u_max  LowerLimit=u_min
  Sum : Sum  Inputs=++|
  Sum1 : Sum  Inputs=++|
  Sum2 : Sum  Inputs=++|
  Sum3 : Sum  Inputs=|+-
  Sum4 : Sum  Inputs=|+-
  u_sat : Outport
  wires:
  Ki/1 -> Integrator/1
  e/1 -> Sum3/1, Kp/1
  e_dot/1 -> Kd/1
  Kp/1 -> Sum/1
  Integrator/1 -> Sum/2
  Sum/1 -> Sum1/2  "u_pi"
  Kd/1 -> Sum1/1
  Sum1/1 -> Sum2/2  "u_pid"
  feedforward/1 -> Sum2/1
  Sum2/1 -> Sum4/1, Saturation/1  "u"
  Saturation/1 -> Sum4/2, u_sat/1
  Sum3/1 -> Ki/1
  Kaw/1 -> Sum3/2
  Sum4/1 -> Kaw/1

== system Simulation/System model/Referenzmodell/Unterlagerte v-Regelung/Unterlagerte Regelung Seil/PT1_Filt ==
  u : Inport
  Integrator : Integrator
  Math Function : Math  Operator=reciprocal  SignedPower=on
  Product : Product
  Sum3 : Sum  Inputs=|+-
  T_filt : Constant  Value=filterMr
  y : Outport  VectorParamsAs1DForOutWhenUnconnected=off
  wires:
  Integrator/1 -> y/1, Sum3/2
  T_filt/1 -> Math Function/1
  u/1 -> Sum3/1
  Product/1 -> Integrator/1
  Sum3/1 -> Product/2
  Math Function/1 -> Product/1

== system Simulation/System model/Referenzmodell/Unterlagerte v-Regelung/Unterlagerte Regelung Wagen/PID AW ==
  e : Inport
  e_dot : Inport  Port=2
  feedforward : Inport  Port=3
  Integrator : Integrator
  Kaw : Gain  Gain=sign(K_I)
  Kd : Gain  Gain=K_D
  Ki : Gain  Gain=K_I
  Kp : Gain  Gain=K_P
  Saturation : Saturate  UpperLimit=u_max  LowerLimit=u_min
  Sum : Sum  Inputs=++|
  Sum1 : Sum  Inputs=++|
  Sum2 : Sum  Inputs=++|
  Sum3 : Sum  Inputs=|+-
  Sum4 : Sum  Inputs=|+-
  u_sat : Outport
  wires:
  Ki/1 -> Integrator/1
  e/1 -> Sum3/1, Kp/1
  e_dot/1 -> Kd/1
  Kp/1 -> Sum/1
  Integrator/1 -> Sum/2
  Sum/1 -> Sum1/2  "u_pi"
  Kd/1 -> Sum1/1
  Sum1/1 -> Sum2/2  "u_pid"
  feedforward/1 -> Sum2/1
  Sum2/1 -> Sum4/1, Saturation/1  "u"
  Saturation/1 -> Sum4/2, u_sat/1
  Sum3/1 -> Ki/1
  Kaw/1 -> Sum3/2
  Sum4/1 -> Kaw/1

== system Simulation/System model/Referenzmodell/Unterlagerte v-Regelung/Unterlagerte Regelung Wagen/PT1_Filt ==
  u : Inport
  Integrator : Integrator
  Math Function : Math  Operator=reciprocal  SignedPower=on
  Product : Product
  Sum3 : Sum  Inputs=|+-
  T_filt : Constant  Value=filterFr
  y : Outport  VectorParamsAs1DForOutWhenUnconnected=off
  wires:
  Integrator/1 -> y/1, Sum3/2
  T_filt/1 -> Math Function/1
  u/1 -> Sum3/1
  Product/1 -> Integrator/1
  Sum3/1 -> Product/2
  Math Function/1 -> Product/1

== system Simulation/System model1/Referenzmodell/Unterlagerte v-Regelung/Unterlagerte Regelung Seil/PID AW ==
  e : Inport
  e_dot : Inport  Port=2
  feedforward : Inport  Port=3
  Integrator : Integrator
  Kaw : Gain  Gain=sign(K_I)
  Kd : Gain  Gain=K_D
  Ki : Gain  Gain=K_I
  Kp : Gain  Gain=K_P
  Saturation : Saturate  UpperLimit=u_max  LowerLimit=u_min
  Sum : Sum  Inputs=++|
  Sum1 : Sum  Inputs=++|
  Sum2 : Sum  Inputs=++|
  Sum3 : Sum  Inputs=|+-
  Sum4 : Sum  Inputs=|+-
  u_sat : Outport
  wires:
  Ki/1 -> Integrator/1
  e/1 -> Sum3/1, Kp/1
  e_dot/1 -> Kd/1
  Kp/1 -> Sum/1
  Integrator/1 -> Sum/2
  Sum/1 -> Sum1/2  "u_pi"
  Kd/1 -> Sum1/1
  Sum1/1 -> Sum2/2  "u_pid"
  feedforward/1 -> Sum2/1
  Sum2/1 -> Sum4/1, Saturation/1  "u"
  Saturation/1 -> Sum4/2, u_sat/1
  Sum3/1 -> Ki/1
  Kaw/1 -> Sum3/2
  Sum4/1 -> Kaw/1

== system Simulation/System model1/Referenzmodell/Unterlagerte v-Regelung/Unterlagerte Regelung Seil/PT1_Filt ==
  u : Inport
  Integrator : Integrator
  Math Function : Math  Operator=reciprocal  SignedPower=on
  Product : Product
  Sum3 : Sum  Inputs=|+-
  T_filt : Constant  Value=filterMr
  y : Outport  VectorParamsAs1DForOutWhenUnconnected=off
  wires:
  Integrator/1 -> y/1, Sum3/2
  T_filt/1 -> Math Function/1
  u/1 -> Sum3/1
  Product/1 -> Integrator/1
  Sum3/1 -> Product/2
  Math Function/1 -> Product/1

== system Simulation/System model1/Referenzmodell/Unterlagerte v-Regelung/Unterlagerte Regelung Wagen/PID AW ==
  e : Inport
  e_dot : Inport  Port=2
  feedforward : Inport  Port=3
  Integrator : Integrator
  Kaw : Gain  Gain=sign(K_I)
  Kd : Gain  Gain=K_D
  Ki : Gain  Gain=K_I
  Kp : Gain  Gain=K_P
  Saturation : Saturate  UpperLimit=u_max  LowerLimit=u_min
  Sum : Sum  Inputs=++|
  Sum1 : Sum  Inputs=++|
  Sum2 : Sum  Inputs=++|
  Sum3 : Sum  Inputs=|+-
  Sum4 : Sum  Inputs=|+-
  u_sat : Outport
  wires:
  Ki/1 -> Integrator/1
  e/1 -> Sum3/1, Kp/1
  e_dot/1 -> Kd/1
  Kp/1 -> Sum/1
  Integrator/1 -> Sum/2
  Sum/1 -> Sum1/2  "u_pi"
  Kd/1 -> Sum1/1
  Sum1/1 -> Sum2/2  "u_pid"
  feedforward/1 -> Sum2/1
  Sum2/1 -> Sum4/1, Saturation/1  "u"
  Saturation/1 -> Sum4/2, u_sat/1
  Sum3/1 -> Ki/1
  Kaw/1 -> Sum3/2
  Sum4/1 -> Kaw/1

== system Simulation/System model1/Referenzmodell/Unterlagerte v-Regelung/Unterlagerte Regelung Wagen/PT1_Filt ==
  u : Inport
  Integrator : Integrator
  Math Function : Math  Operator=reciprocal  SignedPower=on
  Product : Product
  Sum3 : Sum  Inputs=|+-
  T_filt : Constant  Value=filterFr
  y : Outport  VectorParamsAs1DForOutWhenUnconnected=off
  wires:
  Integrator/1 -> y/1, Sum3/2
  T_filt/1 -> Math Function/1
  u/1 -> Sum3/1
  Product/1 -> Integrator/1
  Sum3/1 -> Product/2
  Math Function/1 -> Product/1

== matlab function Simulation/Flatness-based control/quasistatic tracking control/Computation of the flat output/MATLAB Function2 ==
  data: x3 input; x5 input; x6 input; ddz1 output; ddz2 output; u1 input; u2 input; g input
function [ddz1, ddz2] = ddz(x3, x5, x6, u1, u2, g)
    ddz1 = sin(x5) * (u2 + u1 * sin(x5) - x3 * x6^2) - g * sin(x5) * cos(x5);
    ddz2 = cos(x5) * (u2 + u1 * sin(x5) - x3 * x6^2) + g * sin(x5)^2;
end

== matlab function Simulation/Flatness-based control/trajectory generators/desired trajectory: Parabola ==
  data: t input; z1_soll output; T input; z10 input; z1T input; a2 input; a1 input; z2_soll output; a0 input
function [z1_soll, z2_soll] = fcn(t, T, z10, z1T, a2, a1, a0)
% Parabola trajectory generator for avoiding obstacles
%
% Eingangsvariablen:
% t:        Current time
% T:        Duration of the trajectory
% z10:      Initial x-coordinate (horizontal position)
% z1T:      Final x-coordinate (horizontal position)
% a2, a1, a0: Coefficients of the parabolic equation z2 = a2*z1^2 + a1*z1 + a0
%
% Ausgangsvariablen:
% z1_soll:  Horizontal trajectory [z1, dz1, ddz1, ...]
% z2_soll:  Vertical trajectory [z2, dz2, ddz2, ...]

% Initialize output variables
z1_soll = zeros(1, 4); % [Position, Velocity, Acceleration, Jerk]
z2_soll = zeros(1, 4);

% Normalize time
tau = t / T; % Scaled time (0 <= tau <= 1)

% Boundary conditions for z1 (horizontal trajectory)
z1_start = z10;
z1_end = z1T;

% Polynomial coefficients for a fifth-order polynomial for z1
P_z1 = [6, -15, 10, 0, 0, 0]; % Scaled polynomial for smooth interpolation

% Compute z1 trajectory and its derivatives
z1_soll(1) = z1_start + (z1_end - z1_start) * polyval(P_z1, tau);
z1_soll(2) = (z1_end - z1_start) * polyval(polyder(P_z1), tau) / T;
z1_soll(3) = (z1_end - z1_start) * polyval(polyder(polyder(P_z1)), tau) / T^2;
z1_soll(4) = (z1_end - z1_start) * polyval(polyder(polyder(polyder(P_z1))), tau) / T^3;

% Compute z2 (vertical trajectory) based on the parabolic equation
z2_soll(1) = a2 * z1_soll(1)^2 + a1 * z1_soll(1) + a0; % Position
z2_soll(2) = 2 * a2 * z1_soll(1) * z1_soll(2) + a1 * z1_soll(2); % Velocity
z2_soll(3) = 2 * a2 * (z1_soll(2)^2 + z1_soll(1) * z1_soll(3)) + a1 * z1_soll(3); % Acceleration
z2_soll(4) = 2 * a2 * (2 * z1_soll(2) * z1_soll(3) + z1_soll(1) * z1_soll(4)) + a1 * z1_soll(4); % Jerk
end

== matlab function Simulation/Flatness-based control/quasistatic tracking control/Tracking controller/Tracking controller v1 for xLoad/MATLAB Function ==
  data: z1_star input; dz1_star input; ddz1_star input; dddz1_star input; d4z1_star input; z1 input; v1 output; dz1 input; ddz1 input; dddz1 input; pX01 input; pX02 input; pX03 input; pX04 input
function v1 = newInput_v1(z1_star, dz1_star, ddz1_star, dddz1_star, d4z1_star, z1, dz1, ddz1, dddz1, pX01, pX02, pX03, pX04)
    v1 = d4z1_star - pX01 * (dddz1 - dddz1_star) - pX02 * (ddz1 - ddz1_star) - pX03 * (dz1 - dz1_star) - pX04 * (z1 - z1_star);
end

== matlab function Simulation/Flatness-based control/quasistatic tracking control/Tracking controller/Tracking controller v2 for yLoad/MATLAB Function ==
  data: z2_star input; dz2_star input; ddz2_star input; dddz2_star input; d4z2_star input; z2 input; v2 output; dz2 input; pY01_QS input; pY02_QS input; dv2 output; ddv2 output
function [v2, dv2, ddv2] = newInput_v2(z2_star, dz2_star, ddz2_star, dddz2_star, d4z2_star, z2, dz2, pY01_QS, pY02_QS)
    v2 = ddz2_star - pY01_QS * (dz2 - dz2_star) - pY02_QS * (z2 - z2_star);
    dv2 = dddz2_star - pY01_QS * (v2 - ddz2_star) - pY02_QS * (dz2 - dz2_star);
    ddv2 = d4z2_star - pY01_QS * (dv2 - dddz2_star) - pY02_QS * (v2 - ddz2_star);
end

== matlab function Simulation/Flatness-based control/quasistatic tracking control/Tracking controller/MATLAB Function ==
  data: ddz1 input; dddz1 input; v1 input; z2 input; u1 output; dz2 input; v2 input; dv2 input; u2 output; ddv2 input
function [u1, u2] = controlInputs(ddz1, dddz1, v1, z2, dz2, v2, dv2, ddv2)
    g = 9.81;
    
    A = (dz2*ddz1 + z2*dddz1)*(v2 - g);
    dA = (v2*ddz1 + dz2*dddz1*2 + z2*v1) * (v2 - g) + (dz2*ddz1 + z2*dddz1) * dv2;
    B = (A - z2*ddz1*dv2) / ((v2 - g)^2);
    dB = ((dA - dz2*ddz1*dv2 - z2*dddz1*dv2 - z2*ddz1*ddv2) * ((v2 - g)^2) ...
        - (A - z2*ddz1*dv2) * 2*(v2 - g)*dv2) ...
        / ((v2 - g)^4);
    x3 = sqrt(z2^2 + (z2*ddz1/(v2 - g))^2);
    dx3 = (2*z2*dz2 + B) / x3;

    u1 = ddz1 - dB;
    u2 = ((2*dz2*dz2 + 2*z2*v2 + dB)*x3...
        - (2*z2*dz2 + B)*dx3)...
        / (x3^2);
end

== matlab function Simulation/System model/Referenzmodell/Unterlagerte v-Regelung/Unterlagerte Regelung Wagen/MATLAB Function2 ==
  data: mu_W_pos input; c_TW_pos input; c_HW_pos input; v_0_pos input; xdt input; Fr output
function Fr = fcn(mu_W_pos, c_TW_pos, c_HW_pos, v_0_pos, xdt)

%     Fr = -(mu_W_pos*xdt +(c_HW_pos-c_TW_pos)*sign(xdt)*exp(-xdt^2/v_0_pos^2) + c_TW_pos*sign(xdt));
    
    Fr = -(mu_W_pos*xdt + c_TW_pos*sign(xdt));

== matlab function Simulation/Flatness-based control/dynamic tracking control/Computation of the flat output/MATLAB Function ==
  data: x1 input; z1 output; z2 output; x3 input; x5 input
function [z1, z2] = z(x1, x3, x5)
    % Compute flat outputs
    z1 = x1 + x3 * sin(x5);
    z2 = x3 * cos(x5);
end

== matlab function Simulation/Flatness-based control/dynamic tracking control/Computation of the flat output/MATLAB Function1 ==
  data: dz1 output; dz2 output; x2 input; x3 input; x4 input; x5 input; x6 input
function [dz1, dz2] = dz(x2, x3, x4, x5, x6)
    dz1 = x2 + x4 * sin(x5) + x3 * x6 * cos(x5);
    dz2 = x4 * cos(x5) - x3 * x6 * sin(x5);
end

== matlab function Simulation/System model/Referenzmodell/Unterlagerte v-Regelung/Unterlagerte Regelung Seil/MATLAB Function7 ==
  data: muT input; c_TT input; c_HT input; omega_0 input; ldt input; Rho input; Mr output
function Mr = fcn(muT, c_TT, c_HT, omega_0, ldt, Rho)


Mr = -(muT*(-ldt/Rho)+c_TT*sign(-ldt/Rho)+(c_HT-c_TT)*sign(-ldt/Rho)*exp((-ldt^2*omega_0^2)/Rho^2));

% Mr = -(muT*(-ldt/Rho));

== matlab function Simulation/Flatness-based control/dynamic tracking control/Computation of the flat output/MATLAB Function2 ==
  data: x3 input; x5 input; ddz1 output; ddz2 output; x6 input; u1 input; u2 input
function [ddz1, ddz2] = ddz(x3, x5, x6, u1, u2)
  g=9.81
    ddz1 = sin(x5) * (u2 + u1 * sin(x5) - x3 * x6^2) - g * sin(x5) * cos(x5);
    ddz2 = cos(x5) * (u2 + u1 * sin(x5) - x3 * x6^2) + g * sin(x5)^2;
end

== matlab function Simulation/Flatness-based control/dynamic tracking control/System extension/MATLAB Function3 ==
  data: x1_ext input; u2_real output; x3 input; x5 input; x6 input; u1_ext input
function u2_real = compute_u2_real(x1_ext, x3, x5, x6, u1_ext)
    u2_real = x1_ext + x3 * x6^2 - u1_ext * sin(x5);
end

== matlab function Simulation/Flatness-based control/dynamic tracking control/Tracking controller/Tracking controller v1 for xLoad/MATLAB Function ==
  data: z1_star input; dz1_star input; ddz1_star input; dddz1_star input; d4z1_star input; z1 input; v1 output; dz1 input; ddz1 input; dddz1 input; pX01 input; pX02 input; pX03 input; pX04 input
function v1 = newInput_v1(z1_star, dz1_star, ddz1_star, dddz1_star, d4z1_star, z1, dz1, ddz1, dddz1, pX01, pX02, pX03, pX04)
    v1 = d4z1_star - pX01 * (dddz1 - dddz1_star) - pX02 * (ddz1 - ddz1_star) - pX03 * (dz1 - dz1_star) - pX04 * (z1 - z1_star);
end

== matlab function Simulation/Flatness-based control/dynamic tracking control/Tracking controller/Tracking controller v2 for yLoad/MATLAB Function ==
  data: z1_star input; dz1_star input; ddz1_star input; dddz1_star input; d4z1_star input; z1 input; v1 output; dz1 input; ddz1 input; dddz1 input; pY01_DYN input; pY02_DYN input; pY03_DYN input; pY04_DYN input
function v1 = newInput_v1(z1_star, dz1_star, ddz1_star, dddz1_star, d4z1_star, z1, dz1, ddz1, dddz1, pY01_DYN, pY02_DYN, pY03_DYN, pY04_DYN)
    v1 = d4z1_star - pY01_DYN * (dddz1 - dddz1_star) - pY02_DYN * (ddz1 - ddz1_star) - pY03_DYN * (dz1 - dz1_star) - pY04_DYN * (z1 - z1_star);
end

== matlab function Simulation/System model/Kinematisches Modell/sys_dgl  ==
  data: x input; u input; dx output
function dx = fcn(x,u)

dx = zeros(length(x), 1);
g = 9.81;

dx(1) = x(2);
dx(2) = u(1);
dx(3) = x(4);
dx(4) = u(2);
dx(5) = x(6);
dx(6) = -((g * sin(x(5)) + cos(x(5))*u(1) + 2 * x(4) * x(6)) / x(3));

== matlab function Simulation/Flatness-based control/dynamic tracking control/Tracking controller/MATLAB Function ==
  data: ddz1 input; dddz1 input; v1 input; z2 input; dz2 input; ddz2 input; u1 output; dddz2 input; v2 input; u2 output
function [u1, u2] = controlInputs(ddz1, dddz1, v1, z2, dz2, ddz2, dddz2, v2)
    g = 9.81;
    
    A = (dz2*ddz1 + z2*dddz1)*(ddz2 - g);
    dA = (ddz2*ddz1 + dz2*dddz1*2 + z2*v1) * (ddz2 - g) + (dz2*ddz1 + z2*dddz1) * dddz2;
    B = (A - z2*ddz1*dddz2) / ((ddz2 - g)^2);
    dB = ((dA - dz2*ddz1*dddz2 - z2*dddz1*dddz2 - z2*ddz1*v2) * ((ddz2 - g)^2) ...
        - (A - z2*ddz1*dddz2) * 2*(ddz2 - g)*dddz2) ...
        / ((ddz2 - g)^4);
    x3 = sqrt(z2^2 + (z2*ddz1/(ddz2 - g))^2);
    dx3 = (2*z2*dz2 + B) / x3;

    u1 = ddz1 - dB;
    u2 = ((2*dz2*dz2 + 2*z2*ddz2 + dB)*x3...
        - (2*z2*dz2 + B)*dx3)...
        / (x3^2);
end

== matlab function Simulation/Flatness-based control1/dynamic tracking control/Computation of the flat output/MATLAB Function ==
  data: x1 input; z1 output; z2 output; x3 input; x5 input
function [z1, z2] = z(x1, x3, x5)
    % Compute flat outputs
    z1 = x1 + x3 * sin(x5);
    z2 = x3 * cos(x5);
end

== matlab function Simulation/Flatness-based control1/dynamic tracking control/Computation of the flat output/MATLAB Function1 ==
  data: dz1 output; dz2 output; x2 input; x3 input; x4 input; x5 input; x6 input
function [dz1, dz2] = dz(x2, x3, x4, x5, x6)
    dz1 = x2 + x4 * sin(x5) + x3 * x6 * cos(x5);
    dz2 = x4 * cos(x5) - x3 * x6 * sin(x5);
end

== matlab function Simulation/Flatness-based control1/dynamic tracking control/Computation of the flat output/MATLAB Function2 ==
  data: x3 input; x5 input; ddz1 output; ddz2 output; x6 input; u1 input; u2 input
function [ddz1, ddz2] = ddz(x3, x5, x6, u1, u2)
  g=9.81
    ddz1 = sin(x5) * (u2 + u1 * sin(x5) - x3 * x6^2) - g * sin(x5) * cos(x5);
    ddz2 = cos(x5) * (u2 + u1 * sin(x5) - x3 * x6^2) + g * sin(x5)^2;
end

== matlab function Simulation/Flatness-based control1/dynamic tracking control/System extension/MATLAB Function3 ==
  data: x1_ext input; u2_real output; x3 input; x5 input; x6 input; u1_ext input
function u2_real = compute_u2_real(x1_ext, x3, x5, x6, u1_ext)
    u2_real = x1_ext + x3 * x6^2 - u1_ext * sin(x5);
end

== matlab function Simulation/Flatness-based control1/dynamic tracking control/Tracking controller/MATLAB Function ==
  data: ddz1 input; dddz1 input; v1 input; z2 input; dz2 input; ddz2 input; u1 output; dddz2 input; v2 input; u2 output
function [u1, u2] = controlInputs(ddz1, dddz1, v1, z2, dz2, ddz2, dddz2, v2)
    g = 9.81;
    
    A = (dz2*ddz1 + z2*dddz1)*(ddz2 - g);
    dA = (ddz2*ddz1 + dz2*dddz1*2 + z2*v1) * (ddz2 - g) + (dz2*ddz1 + z2*dddz1) * dddz2;
    B = (A - z2*ddz1*dddz2) / ((ddz2 - g)^2);
    dB = ((dA - dz2*ddz1*dddz2 - z2*dddz1*dddz2 - z2*ddz1*v2) * ((ddz2 - g)^2) ...
        - (A - z2*ddz1*dddz2) * 2*(ddz2 - g)*dddz2) ...
        / ((ddz2 - g)^4);
    x3 = sqrt(z2^2 + (z2*ddz1/(ddz2 - g))^2);
    dx3 = (2*z2*dz2 + B) / x3;

    u1 = ddz1 - dB;
    u2 = ((2*dz2*dz2 + 2*z2*ddz2 + dB)*x3...
        - (2*z2*dz2 + B)*dx3)...
        / (x3^2);
end

== matlab function Simulation/Flatness-based control1/dynamic tracking control/Tracking controller/Tracking controller v1 for xLoad/MATLAB Function ==
  data: z1_star input; dz1_star input; ddz1_star input; dddz1_star input; d4z1_star input; z1 input; v1 output; dz1 input; ddz1 input; dddz1 input; pX01 input; pX02 input; pX03 input; pX04 input
function v1 = newInput_v1(z1_star, dz1_star, ddz1_star, dddz1_star, d4z1_star, z1, dz1, ddz1, dddz1, pX01, pX02, pX03, pX04)
    v1 = d4z1_star - pX01 * (dddz1 - dddz1_star) - pX02 * (ddz1 - ddz1_star) - pX03 * (dz1 - dz1_star) - pX04 * (z1 - z1_star);
end

== matlab function Simulation/Plot/yL_Beschraenkung (Parabel) ==
  data: xL input; yL_const output; p0 input; p1 input; p2 input
function yL_const  = fcn(xL, p0, p1, p2)
    % Quadratisches Polynom für die Zustandsbeschränkung p2*x^2+p1*x+p0 (im Horner Schema)
    yL_const = xL * ( p1 + (p2 * xL)) + p0;

end

== matlab function Simulation/Flatness-based control1/dynamic tracking control/Tracking controller/Tracking controller v2 for yLoad/MATLAB Function ==
  data: z1_star input; dz1_star input; ddz1_star input; dddz1_star input; d4z1_star input; z1 input; v1 output; dz1 input; ddz1 input; dddz1 input; pY01_DYN input; pY02_DYN input; pY03_DYN input; pY04_DYN input
function v1 = newInput_v1(z1_star, dz1_star, ddz1_star, dddz1_star, d4z1_star, z1, dz1, ddz1, dddz1, pY01_DYN, pY02_DYN, pY03_DYN, pY04_DYN)
    v1 = d4z1_star - pY01_DYN * (dddz1 - dddz1_star) - pY02_DYN * (ddz1 - ddz1_star) - pY03_DYN * (dz1 - dz1_star) - pY04_DYN * (z1 - z1_star);
end
